simulink model "data_analysis_workspace"  (Simulink 8.6)
settings: Solver=ode45  StartTime=0.0  StopTime=20  RelTol=1e-3
libraries: powerlib_extras x5, powerlib_meascontrol x2, powerlib x1
settings Model: Creator=keliang  LastModifiedBy=Think
settings DataIOCC: SignalLoggingSaveFormat=Dataset
settings OptimizationCC: ExpressionDepthLimit=128  EfficientMapNaN2IntZero=off
settings DebuggingCC: UnderspecifiedInitializationDetection=Simplified  MergeDetectMultiDrivingBlocksExec=error  SolverPrmCheckMsg=none  FcnCallInpInsideContextMsg=EnableAllAsError  StateNameClashWarn=none
settings HardwareCC: ProdBitPerPointer=64  ProdLargestAtomicFloat=Float  ProdIntDivRoundTo=Zero  ProdEndianess=LittleEndian  ProdWordSize=64  ProdHWDeviceType=Intel->x86-64 (Windows64)  TargetBitPerPointer=64  TargetLongLongMode=on  TargetIntDivRoundTo=Zero  TargetEndianess=LittleEndian  TargetWordSize=64  TargetHWDeviceType=MATLAB Host  ProdEqTarget=off
settings CodeAppCC: MaxIdLength=128
settings GRTTargetCC: GeneratePreprocessorConditionals=Use local settings

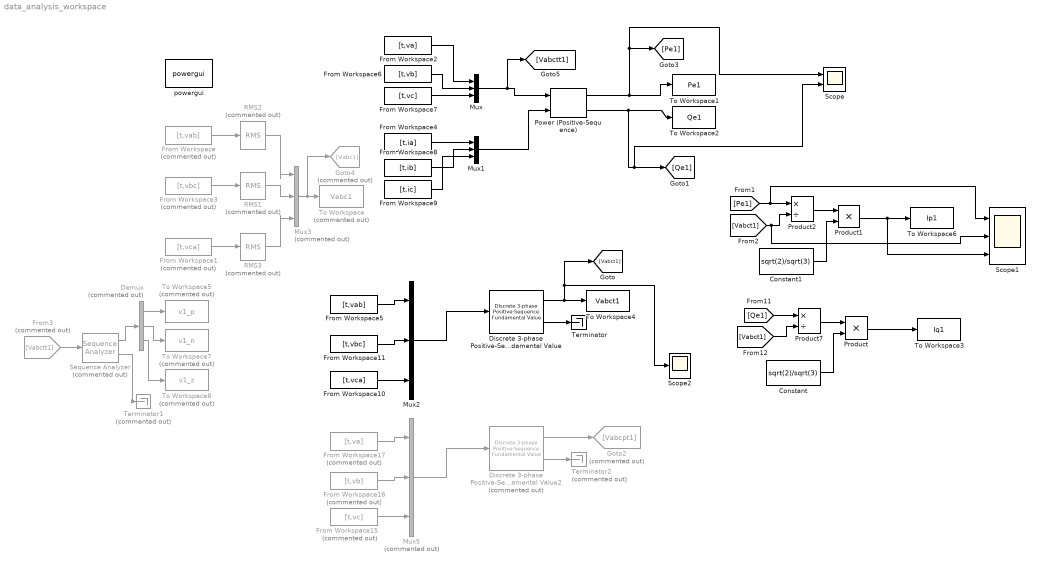
== system data_analysis_workspace ==
  Constant : Constant  Value=sqrt(2)/sqrt(3)
  Constant1 : Constant  Value=sqrt(2)/sqrt(3)
  Demux : Demux  Commented=on  Outputs=3
  Discrete 3-phase Positive-Sequence Fundamental Value : powerlib_extras/Discrete Measurements/Discrete 3-phase Positive-Sequence Fundamental Value  Freq=50  Par_Init=[0 0]  Ts=1e-4
  Discrete 3-phase Positive-Sequence Fundamental Value2 : powerlib_extras/Discrete Measurements/Discrete 3-phase Positive-Sequence Fundamental Value  Commented=on  Freq=50  Par_Init=[0 0]  Ts=1e-4
  From Workspace : FromWorkspace  Commented=on  VariableName=[t,vab]  SampleTime=0
  From Workspace1 : FromWorkspace  Commented=on  VariableName=[t,vca]  SampleTime=0
  From Workspace10 : FromWorkspace  VariableName=[t,vca]  SampleTime=0
  From Workspace11 : FromWorkspace  VariableName=[t,vbc]  SampleTime=0
  From Workspace15 : FromWorkspace  Commented=on  VariableName=[t,vc]  SampleTime=0
  From Workspace16 : FromWorkspace  Commented=on  VariableName=[t,vb]  SampleTime=0
  From Workspace17 : FromWorkspace  Commented=on  VariableName=[t,va]  SampleTime=0
  From Workspace2 : FromWorkspace  VariableName=[t,va]  SampleTime=0
  From Workspace3 : FromWorkspace  Commented=on  VariableName=[t,vbc]  SampleTime=0
  From Workspace4 : FromWorkspace  VariableName=[t,ia]  SampleTime=0
  From Workspace5 : FromWorkspace  VariableName=[t,vab]  SampleTime=0
  From Workspace6 : FromWorkspace  VariableName=[t,vb]  SampleTime=0
  From Workspace7 : FromWorkspace  VariableName=[t,vc]  SampleTime=0
  From Workspace8 : FromWorkspace  VariableName=[t,ib]  SampleTime=0
  From Workspace9 : FromWorkspace  VariableName=[t,ic]  SampleTime=0
  From3 : From  Commented=on  GotoTag=Vabctt1
      settings: CloseFcn=tagdialog Close
  Goto2 : Goto  Commented=on  GotoTag=Vabcpt1
  Goto4 : Goto  Commented=on  GotoTag=Vabc1
  Mux : Mux  Inputs=3
  Mux1 : Mux  Inputs=3
  Mux2 : Mux  Inputs=3
  Mux3 : Mux  Commented=on  Inputs=3
  Mux5 : Mux  Commented=on  Inputs=3
  Power (Positive-Sequence) : powerlib_meascontrol/Measurements/Power (Positive-Sequence)  Freq=50  Vinit=[0, 0]  Iinit=[0, 0]  Ts=0
  Product : Product
  Product1 : Product
  Product2 : Product  Inputs=*/  RndMeth=Zero
  Product7 : Product  Inputs=*/  RndMeth=Zero
  RMS1 : powerlib_extras/Measurements/RMS  Commented=on  f1=50
  RMS2 : powerlib_extras/Measurements/RMS  Commented=on  f1=50
  RMS3 : powerlib_extras/Measurements/RMS  Commented=on  f1=50
  Scope : Scope  NumInputPorts=2
  Scope1 : Scope  NumInputPorts=3
  Scope2 : Scope
  Sequence Analyzer : powerlib_meascontrol/Measurements/Sequence Analyzer  Commented=on  Freq=50  n=1  seq=Positive Negative Zero  InInit=[1, 0]  Ts=0
  Terminator : Terminator
  Terminator1 : Terminator  Commented=on
  Terminator2 : Terminator  Commented=on
  To Workspace : ToWorkspace  Commented=on  VariableName=Vabc1  SaveFormat=Structure With Time  SampleTime=-1
  To Workspace1 : ToWorkspace  VariableName=Pe1  SaveFormat=Structure With Time  SampleTime=-1
  To Workspace2 : ToWorkspace  VariableName=Qe1  SaveFormat=Structure With Time  SampleTime=-1
  To Workspace3 : ToWorkspace  VariableName=Iq1  SaveFormat=Structure With Time  SampleTime=-1
  To Workspace4 : ToWorkspace  VariableName=Vabct1  SaveFormat=Structure With Time  SampleTime=-1
  To Workspace5 : ToWorkspace  Commented=on  VariableName=v1_p  SaveFormat=Structure With Time  SampleTime=-1
  To Workspace6 : ToWorkspace  VariableName=Ip1  SaveFormat=Structure With Time  SampleTime=-1
  To Workspace7 : ToWorkspace  Commented=on  VariableName=v1_n  SaveFormat=Structure With Time  SampleTime=-1
  To Workspace8 : ToWorkspace  Commented=on  VariableName=v1_z  SaveFormat=Structure With Time  SampleTime=-1
  powergui : powerlib/powergui  Priority=1  SimulationMode=Discrete  SolverType=Tustin  SampleTime=20e-6  frequency=60  SPID=off  DisableSnubberDevices=off  DisableRonSwitches=off  DisableVfSwitches=off  SwTol=0  DisplayEquations=off  Interpol=off  ExternalGateDelay=off  methode=off  Ts=10  FunctionMessages=off  echomessages=off  HookPort=off  EnableUseOfTLC=off  x0status=blocks  frequencyindice=60  Pbase=100e6  ErrMax=1e-4  Iterations=50  UnitsV=kV  UnitsW=MW  buscounter=0  RestoreLinks=warning  ResistiveCurrentMeasurement=off  Frange=[0:2:500]  Ylog=off  Xlog=on  ShowGrid=off  save=off  variable=ZData  structure=v1  ZoomFFT=off  StartTime=3  cycles=50  DisplayStyle=1  fundamental=50  FreqAxis=off  MaxFrequency=2000  frequencyindicesteady=1  RmsSteady=1  display=off
  wires:
  From Workspace/1 -> RMS2/1
  From Workspace3/1 -> RMS1/1
  From Workspace1/1 -> RMS3/1
  Power (Positive-Sequence)/1 -> Scope/1, [Pe1], To Workspace1/1
  Power (Positive-Sequence)/2 -> Scope/2, [Qe1], To Workspace2/1
  [Qe1] -> Product7/1
  [Vabct1] -> Product7/2
  Product7/1 -> Product/1
  Constant/1 -> Product/2
  Product/1 -> To Workspace3/1
  Discrete 3-phase Positive-Sequence Fundamental Value/2 -> Terminator/1
  Discrete 3-phase Positive-Sequence Fundamental Value/1 -> Scope2/1, [Vabct1], To Workspace4/1
  Mux/1 -> [Vabctt1], Power (Positive-Sequence)/1
  Mux1/1 -> Power (Positive-Sequence)/2
  From Workspace2/1 -> Mux/1
  From Workspace6/1 -> Mux/2
  From Workspace7/1 -> Mux/3
  From Workspace4/1 -> Mux1/1
  From Workspace8/1 -> Mux1/2
  From Workspace9/1 -> Mux1/3
  From Workspace5/1 -> Mux2/1
  From Workspace11/1 -> Mux2/2
  From Workspace10/1 -> Mux2/3
  Mux2/1 -> Discrete 3-phase Positive-Sequence Fundamental Value/1
  RMS2/1 -> Mux3/1
  RMS1/1 -> Mux3/2
  RMS3/1 -> Mux3/3
  Mux3/1 -> Goto4/1, To Workspace/1
  Discrete 3-phase Positive-Sequence Fundamental Value2/2 -> Terminator2/1
  Discrete 3-phase Positive-Sequence Fundamental Value2/1 -> Goto2/1
  From Workspace17/1 -> Mux5/1
  From Workspace16/1 -> Mux5/2
  From Workspace15/1 -> Mux5/3
  Mux5/1 -> Discrete 3-phase Positive-Sequence Fundamental Value2/1
  [Pe1] -> Scope1/1, Product2/1
  [Vabct1] -> Scope1/2, Product2/2
  Product2/1 -> Product1/1
  Constant1/1 -> Product1/2
  Product1/1 -> Scope1/3, To Workspace6/1
  Sequence Analyzer/1 -> Demux/1
  Demux/1 -> To Workspace5/1
  Demux/2 -> To Workspace7/1
  Demux/3 -> To Workspace8/1
  Sequence Analyzer/2 -> Terminator1/1
  From3/1 -> Sequence Analyzer/1
